simulink model "Linearization2"  (R2022a)
settings: Solver=VariableStepAuto  StartTime=0.0  StopTime=10.0  RelTol=1e-3
undefined symbols (not defined in the file): Aactuator, ac, AeroCoeff, ControlAllocation, DUmax, DUmin, EngineTable, F, fcs, ft, g, hground, IC, kg, LandingGear, Light, LPmethod, m, MIL, Mode_deflection_aileron, Mode_deflection_elevator, Mode_deflection_rudder, Mode_deflection_TVC_y, Mode_deflection_TVC_z, N, Ninv_2nozzle, Ninv_no_nozzle, PIController, s, Sensor, slug, state0, sysID_DAQ, sysID_OBES, Umax_2nozzle, Umax_no_nozzle, Umin_2nozzle, Umin_no_nozzle, WMM2020
libraries: aerolibconvert2 x19, slpidlib x6, simulink x6, sharedutil x4, aerolibatmos2 x3, aerolibwind2 x3, aerolibbdyn x3, aerolibgravity2 x2, sharedtransform x1
(part 8 of 9)

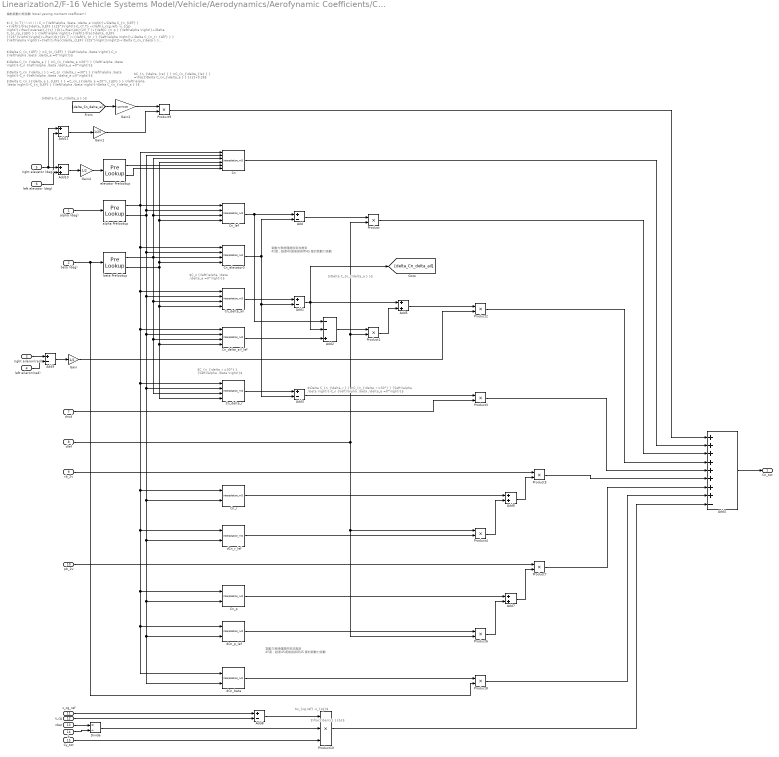
== system Linearization2/F-16 Vehicle Systems Model/Vehicle/Aerodynamics/Aerofynamic Coefficients/CnT ==
  note: $\Delta C_{n_{\delta_a } }$
  note: 氣動力表格僅提供到攻角到
      | 45度，超過45度後皆採用45
      | 度的氣動力係數
  note: 氣動力表格僅提供到攻角到
      | 45度，超過45度後皆採用45
      | 度的氣動力係數
  note: $C_n {\left(\alpha ,\beta ,\delta_e =0°\right)}$
  note: $C_{n_{\delta_r =30°} } {\left(\alpha ,\beta \right)}$
  note: $\Delta C_{n_{\delta_r } } =C_{n_{\delta_r =30°} } {\left(\alpha ,\beta \right)}-C_n {\left(\alpha ,\beta ,\delta_e =0°\right)}$
  note: $x_{cg,ref} -x_{cg}$
  note: $\frac{\bar{c} }{b}$
  note: $\Delta C_{n_{\delta_a } } =C_{n_{\delta_a =20°} } {\left(\alpha ,\beta \right)}-C_n {\left(\alpha ,\beta ,\delta_e =0°\right)}$
  note: $\Delta C_{n_{\delta_r } } =C_{n_{\delta_r =30°} } {\left(\alpha ,\beta \right)}-C_n {\left(\alpha ,\beta ,\delta_e =0°\right)}$
  note: $\ C_{n,T} \ \ =\ \ \ \ C_n {\left(\alpha ,\beta ,\delta_e \right)}+\Delta C_{n_{LEF} } ∙{\left(1-\frac{\delta_{LEF} }{25°}\right)}-C_{Y,T} ∙{\left(x_{cg,ref} -x_{cg} \right)}∙\frac{\overset{-}{c} }{b}+\frac{pb}{2V_T }∙{\left[C_{n_p } {\left(\alpha \right)}+\Delta C_{n_{p_{LEF} } } {\left(\alpha \right)}∙{\left(1-\frac{\delta_{LEF} }{25°}\right)}\right]}+\frac{rb}{2V_T }∙{\left[C_{n_r } {\left(\alpha \right)}+\Delta C_{n_{r_{LEF} } } {\left(\alpha \right)}∙{\left(1-\frac{\delta_{LEF} }{25°}\right)}\right]}+\Delta C_{n_{\beta } } {\left(\alpha \right)}∙\beta +\Delta C_{n_{\delta_r } } ∙{\left(\frac{\delta_r }{30°}\right)}+\frac{{\left[\Delta C_{n_{\delta_a } } +\Delta C_{n_{{\delta_a }_{LEF} } } ∙{\left(1-\frac{\delta_{LEF} }{25°}\right)}\right]}}{2}∙{\left(\frac{\delta_{ra} }{20°}\right)}-\frac{{\left[\Delta C_{n_{\delta_a } } +\Delta C_{n_{{\delta_a }_{LEF} } } ∙{\left(1-\frac{\delta_{LEF} }{25°}\right)}\right]}}{2}∙{\left(\frac{\delta_{la} }{20°}\right)}+C_{n_{\delta_{re} } } ∙{\left(\frac{\delta_{re} }{30°}\right)}-C_{n_{\delta_{le} } } ∙{\left(\frac{\delta_{le} }{30°}\right)}$
  note: $\Delta C_{n_{LEF} } =C_{n_{LEF} } {\left(\alpha ,\beta \right)}-C_n {\left(\alpha ,\beta ,\delta_e =0°\right)}$
  note: 偏航氣動力矩係數 (total yawing moment coefficient)：
  note: $\Delta C_{n_{{\delta_a }_{LEF} } } =C_{n_{{\delta_a =20°}_{LEF} } } {\left(\alpha ,\beta \right)}-C_{n_{LEF} } {\left(\alpha ,\beta \right)}-\Delta C_{n_{\delta_a } }$
  note: $\Delta C_{n_{\delta_a } }$
  note: $C_{n_{\delta_{re} } } =C_{n_{\delta_{le} } } =\frac{\Delta C_{n_{\delta_a } } }{2}∙0.26$
  alpha (deg) : Inport
  beta (deg) : Inport  Port=2
  right aileron(rad) : Inport  Port=3
  left aileron(rad) : Inport  Port=4
  "right elevator (deg) " : Inport  Port=5
  left elevator (deg) : Inport  Port=6
  drud : Inport  Port=7
  dlef : Inport  Port=8
  rb_2v : Inport  Port=9
  pb_2v : Inport  Port=10
  x_cg_ref : Inport  Port=11
  x_cg : Inport  Port=12
  cbar : Inport  Port=13
  b : Inport  Port=14
  Cy_tot : Inport  Port=15
  Add{,1,3,8..9,11} (6 alike) : Sum  Inputs=+-
  Add{5..7,10} (4 alike) : Sum
  Add2 : Sum  Inputs=--+
  Add4 : Sum  Inputs=++++++++-
  Cn : Interpolation_n-D  NumberOfTableDimensions=3  Table=AeroCoeff.Cn
      settings: InputPortMap=u0,u1,u2,u3,u4,u5
  Cn_delta_ail : Interpolation_n-D  Table=AeroCoeff.Cn_delta_ail
  Cn_delta_ail_lef : Interpolation_n-D  Table=AeroCoeff.Cn_delta_ail_lef
  Cn_delta_r : Interpolation_n-D  Table=AeroCoeff.Cn_delta_r
  Cn_elevator0 : Interpolation_n-D  Table=AeroCoeff.Cn_elevator0
  Cn_lef : Interpolation_n-D  Table=AeroCoeff.Cn_lef
  Cn_p : Interpolation_n-D  NumberOfTableDimensions=1  Table=AeroCoeff.Cn_p
      settings: InputPortMap=u0,u1
  Cn_r : Interpolation_n-D  NumberOfTableDimensions=1  Table=AeroCoeff.Cn_r
      settings: InputPortMap=u0,u1
  Divide : Product  Inputs=*/
  Gain : Gain  Gain=1/2
  Gain1 : Gain  Gain=1/25
  Gain2 : Gain  Gain=(1/2)*0.26
  Gain4 : Gain  Gain=1/2
  Product{,1..9} (10 alike) : Product
  Product10 : Product  Inputs=3
  alpha Prelookup : PreLookup  BreakpointsData=AeroCoeff.alpha_prelookup  IndexSearchMethod=Linear search  BeginIndexSearchUsingPreviousIndexResult=on  DiagnosticForOutOfRangeInput=Warning
  beta Prelookup : PreLookup  BreakpointsData=AeroCoeff.beta_prelookup  IndexSearchMethod=Linear search  BeginIndexSearchUsingPreviousIndexResult=on  DiagnosticForOutOfRangeInput=Warning
  dCn_beta : Interpolation_n-D  NumberOfTableDimensions=1  Table=AeroCoeff.dCn_beta
      settings: InputPortMap=u0,u1
  dCn_p_lef : Interpolation_n-D  NumberOfTableDimensions=1  Table=AeroCoeff.dCn_p_lef
      settings: InputPortMap=u0,u1
  dCn_r_lef : Interpolation_n-D  NumberOfTableDimensions=1  Table=AeroCoeff.dCn_r_lef
      settings: InputPortMap=u0,u1
  elevator Prelookup : PreLookup  BreakpointsData=AeroCoeff.elevator_prelookup1  IndexSearchMethod=Linear search  BeginIndexSearchUsingPreviousIndexResult=on  DiagnosticForOutOfRangeInput=Warning
  Cn_tot : Outport  VectorParamsAs1DForOutWhenUnconnected=off
  wires:
  alpha Prelookup/1 -> Cn/1, dCn_p_lef/1, dCn_beta/1, Cn_p/1, dCn_r_lef/1, Cn_r/1, Cn_delta_r/1, Cn_delta_ail_lef/1, Cn_delta_ail/1, Cn_elevator0/1, Cn_lef/1
  Add1/1 -> Add5/1, [delta_Cn_delta_ail], Add2/2
  Cn_elevator0/1 -> Add3/2, Add1/2, Add/2
  alpha Prelookup/2 -> Cn/2, Cn_lef/2, dCn_p_lef/2, dCn_beta/2, Cn_p/2, dCn_r_lef/2, Cn_r/2, Cn_delta_r/2, Cn_delta_ail_lef/2, Cn_delta_ail/2, Cn_elevator0/2
  elevator Prelookup/1 -> Cn/5
  Add6/1 -> Product5/2
  beta Prelookup/2 -> Cn_delta_r/4, Cn_delta_ail_lef/4, Cn_delta_ail/4, Cn/4, Cn_lef/4, Cn_elevator0/4
  Cn_r/1 -> Add6/1
  Cn_delta_ail_lef/1 -> Add2/3
  pb_2v/1 -> Product7/1
  Add5/1 -> Product2/1
  Cn_lef/1 -> Add2/1, Add/1
  Add4/1 -> Cn_tot/1
  Add7/1 -> Product7/2
  beta (deg)/1 -> beta Prelookup/1, Product8/2
  rb_2v/1 -> Product5/1
  Product10/1 -> Add4/9
  Add/1 -> Product/1
  x_cg/1 -> Add8/2
  alpha (deg)/1 -> alpha Prelookup/1
  b/1 -> Divide/2
  dCn_r_lef/1 -> Product4/2
  drud/1 -> Product3/2
  dCn_beta/1 -> Product8/1
  Product4/1 -> Add6/2
  Divide/1 -> Product10/2
  Product3/1 -> Add4/5
  x_cg_ref/1 -> Add8/1
  Cn_p/1 -> Add7/1
  dCn_p_lef/1 -> Product6/1
  Product8/1 -> Add4/8
  elevator Prelookup/2 -> Cn/6
  Cn_delta_r/1 -> Add3/1
  Product6/1 -> Add7/2
  Cy_tot/1 -> Product10/3
  Product7/1 -> Add4/7
  Product5/1 -> Add4/6
  Add2/1 -> Product1/1
  beta Prelookup/1 -> Cn_delta_r/3, Cn_delta_ail_lef/3, Cn_delta_ail/3, Cn/3, Cn_lef/3, Cn_elevator0/3
  Product2/1 -> Add4/4
  Cn/1 -> Add4/2
  Cn_delta_ail/1 -> Add1/1
  Add3/1 -> Product3/1
  dlef/1 -> Product6/2, Product4/1, Product/2, Product1/2
  Product/1 -> Add4/3
  Product1/1 -> Add5/2
  cbar/1 -> Divide/1
  Add8/1 -> Product10/1
  right aileron(rad)/1 -> Add9/1
  left aileron(rad)/1 -> Add9/2
  Add9/1 -> Gain/1
  Gain/1 -> Product2/2
  Add10/1 -> Gain4/1
  [delta_Cn_delta_ail] -> Gain2/1
  Gain1/1 -> Product9/2
  Gain2/1 -> Product9/1
  Product9/1 -> Add4/1
  "right elevator (deg) "/1 -> Add11/1, Add10/1
  left elevator (deg)/1 -> Add11/2, Add10/2
  Add11/1 -> Gain1/1
  Gain4/1 -> elevator Prelookup/1

== system Linearization2/F-16 Vehicle Systems Model/Vehicle/Aerodynamics/Aerofynamic Coefficients/Ground Effects ==
  alpha (deg) : Inport
  beta(deg) : Inport  Port=2
  h_AGL : Inport  Port=3
  Coeff : Outport

== system Linearization2/F-16 Vehicle Systems Model/Vehicle/Aerodynamics/Aerofynamic Coefficients/Landing Gear Effects ==
  alpha (deg) : Inport
  beta(deg) : Inport  Port=2
  Landing Gear Angle : Inport  Port=3
  Coeff : Outport

== system Linearization2/F-16 Vehicle Systems Model/Vehicle/LandingGear GroundReaction/L Main Gear Geometry Forces and Moments/Calc Gear Force and Pos ==
  note: 註:令[ XcB YcB ZcB ] = [ 0 0 0 ]
  note: 詹庭宇:此Block正負號為+---
  note: $∆z_g^B$
  note: $∆z_g^b =z_g^b -z_g^{b^{\prime } } =z_g^b -\frac{z_r^E -z_c^E -C_{31} {\left(x_g^b -x_c^b \right)}-C_{32} {\left(y_g^b -y_c^b \right)}}{C_{33} }$
  note: $z_r^E =z_c^E +C_{31} {\left(x_g^b -x_c^b \right)}+C_{32} {\left(y_g^b -y_c^b \right)}+C_{33} \cdot z_g^{b^{\prime } }$
  note: $z_g^E =z_c^E +C_{31} {\left(x_g^b -x_c^b \right)}+C_{32} {\left(y_g^b -y_c^b \right)}+C_{33} {\left(z_g^b -z_c^b \right)}$
  note: $p^E ={\left[C\right]}{\left(p^b -p_c^b \right)}+p_c^E$
  note: $\left(p^E -p_c^E \right)={\left[C\right]}{\left(p^b -p_c^b \right)}$
  note: 定義：
      | 慣性座標+Z軸朝下
      | 體座標+Z軸朝下
  WOW : Inport
  ZrL : Inport  Port=2
  Xg : Inport  Port=3
  ZcL : Inport  Port=4
  DCM_eb : Inport  Port=5
  Constant : Constant  Value=0
  Demux1 : Demux  Outputs=3
  Demux2 : Demux  Outputs=3
  RangeLimit : Saturate  UpperLimit=LandingGear.LM.CmprsRangeLimitUpper  LowerLimit=LandingGear.LM.CmprsRangeLimitLower
  Subsystem : Subsystem
  Sum1 : Sum  Inputs=+---
  Sum2 : Sum  Inputs=+-
  Switch : Switch  Criteria=u2 ~= 0  Threshold=243  SaturateOnIntegerOverflow=off  InputSameDT=off
  compression : Product  Inputs=*/  RndMeth=Zero
  get_row3 : Selector  NumberOfDimensions=2  InputPortWidth=3  IndexOptions=Index vector (dialog),Select all  Indices=3,-1  OutputSizes=1
  prod1 : Product  RndMeth=Zero
  prod2 : Product  RndMeth=Zero
  dZ_strut : Outport
  Fn_strut : Outport  Port=2
  ZgB_prime : Outport  Port=3
  wires:
  ZrL/1 -> Sum1/1
  DCM_eb/1 -> get_row3/1
  get_row3/1 -> Demux1/1  "C3"
  Demux1/1 -> prod1/2  "C31"
  Demux1/2 -> prod2/2  "C32"
  Demux2/1 -> prod1/1  "XgB-XcB"
  Demux2/2 -> prod2/1  "YgB-YcB"
  prod1/1 -> Sum1/3
  prod2/1 -> Sum1/4
  Demux1/3 -> compression/2, Subsystem/2(C33)  "C33"
  Subsystem/2(Fn_strut) -> Fn_strut/1
  compression/1 -> Sum2/2, ZgB_prime/1
  ZcL/1 -> Sum1/2
  Xg/1 -> Demux2/1
  Sum1/1 -> compression/1  "Strut_dZnum"
  Demux2/3 -> Sum2/1  "ZgB-ZcB"
  Subsystem/1(dZ_strut) -> dZ_strut/1
  RangeLimit/1 -> Subsystem/1(deltaZgB)
  Switch/1 -> RangeLimit/1
  Sum2/1 -> Switch/1  "T command"
  WOW/1 -> Switch/2
  Constant/1 -> Switch/3  "T command"

== system Linearization2/F-16 Vehicle Systems Model/Vehicle/LandingGear GroundReaction/L Main Gear Geometry Forces and Moments/GenerateGroundFM ==
  note: 正負號可能相反
  note: 慣性座標轉至體座標的旋轉矩陣
  note: 詹庭宇:拿掉/忽略輪胎側向力模型，Fy=0
  note: 詹庭宇:拿掉/忽略輪胎側向力模型，Fy=0
  GearLoc : Inport
  Fn_strut : Inport  Port=2
  ZgB_prime : Inport  Port=3
  DCM_be : Inport  Port=4
  plant : Inport  Port=5
  Enable : EnablePort
  Constant : Constant  Value=0
  Constant1 : Constant  Value=[0 0 0]
  Demux : Demux  Outputs=3
  Forces and distances to LMN : Subsystem
  Gear Local Force vector : Concatenate  NumInputs=3  Mode=Multidimensional array
  LocMatrix1 : Subsystem
  Local Forces to Body Axes : Product  Multiplication=Matrix(*)  InputSameDT=on  SaturateOnIntegerOverflow=on  OutDataTypeStr=Inherit: Same as first input
  Manual Switch : ManualSwitch  CurrentSetting=0
  Moments about CG due to Forces : aerolibbdyn/Moments about CG  due to Forces
      settings: SourceProductBaseCode=AE
  Mux1 : Mux  Inputs=2
  Mux2 : Mux  Inputs=3
  Rotation Speed(TVC ON) : Subsystem
  Terminator : Terminator
  FM : Outport
  wires:
  DCM_be/1 -> Local Forces to Body Axes/1
  Mux1/1 -> FM/1
  Local Forces to Body Axes/1 -> Moments about CG due to Forces/1, Forces and distances to LMN/1(Fb)
  Gear Local Force vector/1 -> Local Forces to Body Axes/2, Mux1/1
  Constant/1 -> Gear Local Force vector/2
  ZgB_prime/1 -> Mux2/3, LocMatrix1/2(ZgB_prime)
  Forces and distances to LMN/1(LMNe) -> Manual Switch/1
  Manual Switch/1 -> Mux1/2
  Moments about CG due to Forces/1 -> Manual Switch/2
  Constant1/1 -> Moments about CG due to Forces/2
  LocMatrix1/1(A) -> Forces and distances to LMN/2(Xg_gnd)
  Demux/1 -> Mux2/1
  Demux/3 -> Terminator/1
  GearLoc/1 -> Demux/1, LocMatrix1/1(XgB)
  Mux2/1 -> Moments about CG due to Forces/3
  Demux/2 -> Mux2/2
  plant/1 -> Rotation Speed(TVC ON)/2(PlantData)
  Fn_strut/1 -> Gear Local Force vector/3, Rotation Speed(TVC ON)/1(friction)
  Rotation Speed(TVC ON)/1(output) -> Gear Local Force vector/1

== system Linearization2/F-16 Vehicle Systems Model/Vehicle/LandingGear GroundReaction/Nose Gear Geometry Forces and Moments/Calc Gear Force and Pos ==
  note: 註:令[ XcB YcB ZcB ] = [ 0 0 0 ]
  note: 詹庭宇:此Block正負號為+---
  note: $∆z_g^B$
  note: $∆z_g^b =z_g^b -z_g^{b^{\prime } } =z_g^b -\frac{z_r^E -z_c^E -C_{31} {\left(x_g^b -x_c^b \right)}-C_{32} {\left(y_g^b -y_c^b \right)}}{C_{33} }$
  note: $z_r^E =z_c^E +C_{31} {\left(x_g^b -x_c^b \right)}+C_{32} {\left(y_g^b -y_c^b \right)}+C_{33} \cdot z_g^{b^{\prime } }$
  note: $z_g^E =z_c^E +C_{31} {\left(x_g^b -x_c^b \right)}+C_{32} {\left(y_g^b -y_c^b \right)}+C_{33} {\left(z_g^b -z_c^b \right)}$
  note: $p^E ={\left[C\right]}{\left(p^b -p_c^b \right)}+p_c^E$
  note: $\left(p^E -p_c^E \right)={\left[C\right]}{\left(p^b -p_c^b \right)}$
  note: 定義：
      | 慣性座標+Z軸朝下
      | 體座標+Z軸朝下
  WOW : Inport
  ZrL : Inport  Port=2
  Xg : Inport  Port=3
  ZcL : Inport  Port=4
  DCM_eb : Inport  Port=5
  Constant : Constant  Value=0
  Demux1 : Demux  Outputs=3
  Demux2 : Demux  Outputs=3
  RangeLimit : Saturate  UpperLimit=LandingGear.Nose.CmprsRangeLimitUpper  LowerLimit=LandingGear.Nose.CmprsRangeLimitLower
  Subsystem : Subsystem
  Sum1 : Sum  Inputs=+---
  Sum2 : Sum  Inputs=+-
  Switch : Switch  Criteria=u2 ~= 0  Threshold=243  SaturateOnIntegerOverflow=off  InputSameDT=off
  compression : Product  Inputs=*/  RndMeth=Zero
  get_row3 : Selector  NumberOfDimensions=2  InputPortWidth=3  IndexOptions=Index vector (dialog),Select all  Indices=3,-1  OutputSizes=1
  prod1 : Product  RndMeth=Zero
  prod2 : Product  RndMeth=Zero
  dZ_strut : Outport
  Fn_strut : Outport  Port=2
  ZgB_prime : Outport  Port=3
  wires:
  ZrL/1 -> Sum1/1
  DCM_eb/1 -> get_row3/1
  get_row3/1 -> Demux1/1  "C3"
  Demux1/1 -> prod1/2  "C31"
  Demux1/2 -> prod2/2  "C32"
  Demux2/1 -> prod1/1  "XgB-XcB"
  Demux2/2 -> prod2/1  "YgB-YcB"
  prod1/1 -> Sum1/3
  prod2/1 -> Sum1/4
  Demux1/3 -> compression/2, Subsystem/2(C33)  "C33"
  Subsystem/2(Fn_strut) -> Fn_strut/1
  compression/1 -> Sum2/2, ZgB_prime/1
  ZcL/1 -> Sum1/2
  Xg/1 -> Demux2/1
  Sum1/1 -> compression/1  "Strut_dZnum"
  Demux2/3 -> Sum2/1  "ZgB-ZcB"
  Subsystem/1(dZ_strut) -> dZ_strut/1
  RangeLimit/1 -> Subsystem/1(deltaZgB)
  Switch/1 -> RangeLimit/1
  Sum2/1 -> Switch/1  "T command"
  WOW/1 -> Switch/2
  Constant/1 -> Switch/3  "T command"

== system Linearization2/F-16 Vehicle Systems Model/Vehicle/LandingGear GroundReaction/Nose Gear Geometry Forces and Moments/GenerateGroundFM ==
  note: 正負號可能相反
  note: 慣性座標轉至體座標的旋轉矩陣
  note: 詹庭宇:拿掉/忽略輪胎側向力模型，Fy=0
  note: 詹庭宇:拿掉/忽略輪胎側向力模型，Fy=0
  GearLoc : Inport
  Fn_strut : Inport  Port=2
  ZgB_prime : Inport  Port=3
  DCM_be : Inport  Port=4
  plant : Inport  Port=5
  Enable : EnablePort
  Constant : Constant  Value=0
  Constant1 : Constant  Value=[0 0 0]
  Demux : Demux  Outputs=3
  Forces and distances to LMN : Subsystem
  Gear Local Force vector : Concatenate  NumInputs=3  Mode=Multidimensional array
  LocMatrix1 : Subsystem
  Local Forces to Body Axes : Product  Multiplication=Matrix(*)  InputSameDT=on  SaturateOnIntegerOverflow=on  OutDataTypeStr=Inherit: Same as first input
  Manual Switch : ManualSwitch  CurrentSetting=0
  Moments about CG due to Forces : aerolibbdyn/Moments about CG  due to Forces
      settings: SourceProductBaseCode=AE
  Mux1 : Mux  Inputs=2
  Mux2 : Mux  Inputs=3
  Rotation Speed(TVC ON) : Subsystem
  Terminator : Terminator
  FM : Outport
  wires:
  DCM_be/1 -> Local Forces to Body Axes/1
  Mux1/1 -> FM/1
  Local Forces to Body Axes/1 -> Moments about CG due to Forces/1, Forces and distances to LMN/1(Fb)
  Gear Local Force vector/1 -> Local Forces to Body Axes/2, Mux1/1
  Constant/1 -> Gear Local Force vector/2
  ZgB_prime/1 -> Mux2/3, LocMatrix1/2(ZgB_prime)
  Forces and distances to LMN/1(LMNe) -> Manual Switch/1
  Manual Switch/1 -> Mux1/2
  Moments about CG due to Forces/1 -> Manual Switch/2
  Constant1/1 -> Moments about CG due to Forces/2
  LocMatrix1/1(A) -> Forces and distances to LMN/2(Xg_gnd)
  Demux/1 -> Mux2/1
  Demux/3 -> Terminator/1
  GearLoc/1 -> Demux/1, LocMatrix1/1(XgB)
  Mux2/1 -> Moments about CG due to Forces/3
  Demux/2 -> Mux2/2
  plant/1 -> Rotation Speed(TVC ON)/2(PlantData)
  Fn_strut/1 -> Gear Local Force vector/3, Rotation Speed(TVC ON)/1(friction)
  Rotation Speed(TVC ON)/1(output) -> Gear Local Force vector/1

== system Linearization2/F-16 Vehicle Systems Model/Vehicle/LandingGear GroundReaction/R Main Gear Geometry Forces and Moments/Calc Gear Force and Pos ==
  note: 註:令[ XcB YcB ZcB ] = [ 0 0 0 ]
  note: 詹庭宇:此Block正負號為+---
  note: $∆z_g^B$
  note: $∆z_g^b =z_g^b -z_g^{b^{\prime } } =z_g^b -\frac{z_r^E -z_c^E -C_{31} {\left(x_g^b -x_c^b \right)}-C_{32} {\left(y_g^b -y_c^b \right)}}{C_{33} }$
  note: $z_r^E =z_c^E +C_{31} {\left(x_g^b -x_c^b \right)}+C_{32} {\left(y_g^b -y_c^b \right)}+C_{33} \cdot z_g^{b^{\prime } }$
  note: $z_g^E =z_c^E +C_{31} {\left(x_g^b -x_c^b \right)}+C_{32} {\left(y_g^b -y_c^b \right)}+C_{33} {\left(z_g^b -z_c^b \right)}$
  note: $p^E ={\left[C\right]}{\left(p^b -p_c^b \right)}+p_c^E$
  note: $\left(p^E -p_c^E \right)={\left[C\right]}{\left(p^b -p_c^b \right)}$
  note: 定義：
      | 慣性座標+Z軸朝下
      | 體座標+Z軸朝下
  WOW : Inport
  ZrL : Inport  Port=2
  Xg : Inport  Port=3
  ZcL : Inport  Port=4
  DCM_eb : Inport  Port=5
  Constant : Constant  Value=0
  Demux1 : Demux  Outputs=3
  Demux2 : Demux  Outputs=3
  RangeLimit : Saturate  UpperLimit=LandingGear.RM.CmprsRangeLimitUpper  LowerLimit=LandingGear.RM.CmprsRangeLimitLower
  Subsystem : Subsystem
  Sum1 : Sum  Inputs=+---
  Sum2 : Sum  Inputs=+-
  Switch : Switch  Criteria=u2 ~= 0  Threshold=243  SaturateOnIntegerOverflow=off  InputSameDT=off
  compression : Product  Inputs=*/  RndMeth=Zero
  get_row3 : Selector  NumberOfDimensions=2  InputPortWidth=3  IndexOptions=Index vector (dialog),Select all  Indices=3,-1  OutputSizes=1
  prod1 : Product  RndMeth=Zero
  prod2 : Product  RndMeth=Zero
  dZ_strut : Outport
  Fn_strut : Outport  Port=2
  ZgB_prime : Outport  Port=3
  wires:
  ZrL/1 -> Sum1/1
  DCM_eb/1 -> get_row3/1
  get_row3/1 -> Demux1/1  "C3"
  Demux1/1 -> prod1/2  "C31"
  Demux1/2 -> prod2/2  "C32"
  Demux2/1 -> prod1/1  "XgB-XcB"
  Demux2/2 -> prod2/1  "YgB-YcB"
  prod1/1 -> Sum1/3
  prod2/1 -> Sum1/4
  Demux1/3 -> compression/2, Subsystem/2(C33)  "C33"
  Subsystem/2(Fn_strut) -> Fn_strut/1
  compression/1 -> Sum2/2, ZgB_prime/1
  ZcL/1 -> Sum1/2
  Xg/1 -> Demux2/1
  Sum1/1 -> compression/1  "Strut_dZnum"
  Demux2/3 -> Sum2/1  "ZgB-ZcB"
  Subsystem/1(dZ_strut) -> dZ_strut/1
  RangeLimit/1 -> Subsystem/1(deltaZgB)
  Switch/1 -> RangeLimit/1
  Sum2/1 -> Switch/1  "T command"
  WOW/1 -> Switch/2
  Constant/1 -> Switch/3  "T command"

== system Linearization2/F-16 Vehicle Systems Model/Vehicle/LandingGear GroundReaction/R Main Gear Geometry Forces and Moments/GenerateGroundFM ==
  note: 正負號可能相反
  note: 慣性座標轉至體座標的旋轉矩陣
  note: 詹庭宇:拿掉/忽略輪胎側向力模型，Fy=0
  note: 詹庭宇:拿掉/忽略輪胎側向力模型，Fy=0
  GearLoc : Inport
  Fn_strut : Inport  Port=2
  ZgB_prime : Inport  Port=3
  DCM_be : Inport  Port=4
  plant : Inport  Port=5
  Enable : EnablePort
  Constant : Constant  Value=0
  Constant1 : Constant  Value=[0 0 0]
  Demux : Demux  Outputs=3
  Forces and distances to LMN : Subsystem
  Gear Local Force vector : Concatenate  NumInputs=3  Mode=Multidimensional array
  LocMatrix1 : Subsystem
  Local Forces to Body Axes : Product  Multiplication=Matrix(*)  InputSameDT=on  SaturateOnIntegerOverflow=on  OutDataTypeStr=Inherit: Same as first input
  Manual Switch : ManualSwitch  CurrentSetting=0
  Moments about CG due to Forces : aerolibbdyn/Moments about CG  due to Forces
      settings: SourceProductBaseCode=AE
  Mux1 : Mux  Inputs=2
  Mux2 : Mux  Inputs=3
  Rotation Speed(TVC ON) : Subsystem
  Terminator : Terminator
  FM : Outport
  wires:
  DCM_be/1 -> Local Forces to Body Axes/1
  Mux1/1 -> FM/1
  Local Forces to Body Axes/1 -> Moments about CG due to Forces/1, Forces and distances to LMN/1(Fb)
  Gear Local Force vector/1 -> Local Forces to Body Axes/2, Mux1/1
  Constant/1 -> Gear Local Force vector/2
  ZgB_prime/1 -> Mux2/3, LocMatrix1/2(ZgB_prime)
  Forces and distances to LMN/1(LMNe) -> Manual Switch/1
  Manual Switch/1 -> Mux1/2
  Moments about CG due to Forces/1 -> Manual Switch/2
  Constant1/1 -> Moments about CG due to Forces/2
  LocMatrix1/1(A) -> Forces and distances to LMN/2(Xg_gnd)
  Demux/1 -> Mux2/1
  Demux/3 -> Terminator/1
  GearLoc/1 -> Demux/1, LocMatrix1/1(XgB)
  Mux2/1 -> Moments about CG due to Forces/3
  Demux/2 -> Mux2/2
  plant/1 -> Rotation Speed(TVC ON)/2(PlantData)
  Fn_strut/1 -> Gear Local Force vector/3, Rotation Speed(TVC ON)/1(friction)
  Rotation Speed(TVC ON)/1(output) -> Gear Local Force vector/1

== system Linearization2/F-16 Vehicle Systems Model/Vehicle/Propulsion/Afterburning Turbofan Jet Engine/If Action Subsystem ==
  note: Pow_max
      |
      | Pow_min
      |
      | T_idle
      |
      | T_mil
      |
      | T_max
  "input " : Inport
  Action Port : ActionPort
  Add : Sum
  Add1 : Sum  Inputs=-+
  Demux : Demux  Outputs=5
  Divide : Product  Inputs=**
  Gain : Gain  Gain=1/50
  Terminator : Terminator
  Terminator1 : Terminator
  T_max1 : Outport  VectorParamsAs1DForOutWhenUnconnected=off
  wires:
  Demux/3 -> Add1/1, Add/1
  Demux/4 -> Add1/2
  Add1/1 -> Divide/2
  Gain/1 -> Divide/1
  Divide/1 -> Add/2
  Add/1 -> T_max1/1
  "input "/1 -> Demux/1
  Demux/1 -> Gain/1
  Demux/2 -> Terminator/1
  Demux/5 -> Terminator1/1

== system Linearization2/F-16 Vehicle Systems Model/Vehicle/Propulsion/Afterburning Turbofan Jet Engine/If Action Subsystem1 ==
  note: Pow_max
      |
      | Pow_min
      |
      | T_idle
      |
      | T_mil
      |
      | T_max
  "input " : Inport
  Action Port : ActionPort
  Add : Sum
  Add1 : Sum  Inputs=-+
  Add2 : Sum  Inputs=-+
  Constant : Constant  Value=50
  Demux : Demux  Outputs=5
  Gain : Gain  Gain=1/50
  Product : Product
  Terminator : Terminator
  Terminator1 : Terminator
  T_max1 : Outport  VectorParamsAs1DForOutWhenUnconnected=off
  wires:
  "input "/1 -> Demux/1
  Demux/4 -> Add/2, Add1/1
  Demux/5 -> Add1/2
  Demux/1 -> Add2/2
  Constant/1 -> Add2/1
  Add2/1 -> Gain/1
  Add1/1 -> Product/2
  Gain/1 -> Product/1
  Product/1 -> Add/1
  Add/1 -> T_max1/1
  Demux/3 -> Terminator1/1
  Demux/2 -> Terminator/1

== system Linearization2/F-16 Vehicle Systems Model/Vehicle/Propulsion/Afterburning Turbofan Jet Engine/If Action Subsystem2 ==
  note: Pow_max
      |
      | Pow_min
      |
      | T_idle
      |
      | T_mil
      |
      | T_max
  "input " : Inport
  Action Port : ActionPort
  Add : Sum
  Add1 : Sum  Inputs=-+
  Demux : Demux  Outputs=5
  Divide : Product  Inputs=**
  Gain : Gain  Gain=1/50
  Terminator : Terminator
  Terminator1 : Terminator
  T_min : Outport  VectorParamsAs1DForOutWhenUnconnected=off
  wires:
  Demux/3 -> Add1/1, Add/1
  Demux/4 -> Add1/2
  Add1/1 -> Divide/2
  Gain/1 -> Divide/1
  Divide/1 -> Add/2
  Add/1 -> T_min/1
  "input "/1 -> Demux/1
  Demux/2 -> Gain/1
  Demux/5 -> Terminator1/1
  Demux/1 -> Terminator/1

== system Linearization2/F-16 Vehicle Systems Model/Vehicle/Propulsion/Afterburning Turbofan Jet Engine/If Action Subsystem3 ==
  note: Pow_max
      |
      | Pow_min
      |
      | T_idle
      |
      | T_mil
      |
      | T_max
  "input " : Inport
  Action Port : ActionPort
  Add : Sum
  Add1 : Sum  Inputs=-+
  Add2 : Sum  Inputs=-+
  Constant : Constant  Value=50
  Demux : Demux  Outputs=5
  Gain : Gain  Gain=1/50
  Product : Product
  Terminator : Terminator
  Terminator1 : Terminator
  T_min : Outport  VectorParamsAs1DForOutWhenUnconnected=off
  wires:
  "input "/1 -> Demux/1
  Demux/4 -> Add/2, Add1/1
  Demux/5 -> Add1/2
  Constant/1 -> Add2/1
  Add2/1 -> Gain/1
  Add1/1 -> Product/2
  Gain/1 -> Product/1
  Product/1 -> Add/1
  Add/1 -> T_min/1
  Demux/3 -> Terminator1/1
  Demux/2 -> Add2/2
  Demux/1 -> Terminator/1

== system Linearization2/F-16 Vehicle Systems Model/Vehicle/Propulsion/Afterburning Turbofan Jet Engine/If Action Subsystem4 ==
  In1 : Inport
  Action Port : ActionPort
  Out1 : Outport
  wires:
  In1/1 -> Out1/1

== system Linearization2/F-16 Vehicle Systems Model/Vehicle/Propulsion/Afterburning Turbofan Jet Engine/If Action Subsystem5 ==
  In1 : Inport
  Action Port : ActionPort
  Out1 : Outport
  wires:
  In1/1 -> Out1/1

== system Linearization2/F-16 Vehicle Systems Model/Vehicle/Propulsion/Afterburning Turbofan Jet Engine/If Action Subsystem6 ==
  In1 : Inport
  Action Port : ActionPort
  Out1 : Outport
  wires:
  In1/1 -> Out1/1

== system Linearization2/F-16 Vehicle Systems Model/Vehicle/Propulsion(two_nozzles)/Afterburning Turbofan Jet Engine/If Action Subsystem ==
  note: Pow_max
      |
      | Pow_min
      |
      | T_idle
      |
      | T_mil
      |
      | T_max
  "input " : Inport
  Action Port : ActionPort  ActionPortLabel=if(u1<50)
  Add : Sum
  Add1 : Sum  Inputs=-+
  Demux : Demux  Outputs=5
  Divide : Product  Inputs=**
  Gain : Gain  Gain=1/50
  Terminator : Terminator
  Terminator1 : Terminator
  T_max1 : Outport  VectorParamsAs1DForOutWhenUnconnected=off
  wires:
  Demux/3 -> Add1/1, Add/1
  Demux/4 -> Add1/2
  Add1/1 -> Divide/2
  Gain/1 -> Divide/1
  Divide/1 -> Add/2
  Add/1 -> T_max1/1
  "input "/1 -> Demux/1
  Demux/1 -> Gain/1
  Demux/2 -> Terminator/1
  Demux/5 -> Terminator1/1

== system Linearization2/F-16 Vehicle Systems Model/Vehicle/Propulsion(two_nozzles)/Afterburning Turbofan Jet Engine/If Action Subsystem1 ==
  note: Pow_max
      |
      | Pow_min
      |
      | T_idle
      |
      | T_mil
      |
      | T_max
  "input " : Inport
  Action Port : ActionPort  ActionPortLabel=elseif(u1>=50)
  Add : Sum
  Add1 : Sum  Inputs=-+
  Add2 : Sum  Inputs=-+
  Constant : Constant  Value=50
  Demux : Demux  Outputs=5
  Gain : Gain  Gain=1/50
  Product : Product
  Terminator : Terminator
  Terminator1 : Terminator
  T_max1 : Outport  VectorParamsAs1DForOutWhenUnconnected=off
  wires:
  "input "/1 -> Demux/1
  Demux/4 -> Add/2, Add1/1
  Demux/5 -> Add1/2
  Demux/1 -> Add2/2
  Constant/1 -> Add2/1
  Add2/1 -> Gain/1
  Add1/1 -> Product/2
  Gain/1 -> Product/1
  Product/1 -> Add/1
  Add/1 -> T_max1/1
  Demux/3 -> Terminator1/1
  Demux/2 -> Terminator/1

== system Linearization2/F-16 Vehicle Systems Model/Vehicle/Propulsion(two_nozzles)/Afterburning Turbofan Jet Engine/If Action Subsystem2 ==
  note: Pow_max
      |
      | Pow_min
      |
      | T_idle
      |
      | T_mil
      |
      | T_max
  "input " : Inport
  Action Port : ActionPort  ActionPortLabel=if(u1<50)
  Add : Sum
  Add1 : Sum  Inputs=-+
  Demux : Demux  Outputs=5
  Divide : Product  Inputs=**
  Gain : Gain  Gain=1/50
  Terminator : Terminator
  Terminator1 : Terminator
  T_min : Outport  VectorParamsAs1DForOutWhenUnconnected=off
  wires:
  Demux/3 -> Add1/1, Add/1
  Demux/4 -> Add1/2
  Add1/1 -> Divide/2
  Gain/1 -> Divide/1
  Divide/1 -> Add/2
  Add/1 -> T_min/1
  "input "/1 -> Demux/1
  Demux/2 -> Gain/1
  Demux/5 -> Terminator1/1
  Demux/1 -> Terminator/1

== system Linearization2/F-16 Vehicle Systems Model/Vehicle/Propulsion(two_nozzles)/Afterburning Turbofan Jet Engine/If Action Subsystem3 ==
  note: Pow_max
      |
      | Pow_min
      |
      | T_idle
      |
      | T_mil
      |
      | T_max
  "input " : Inport
  Action Port : ActionPort  ActionPortLabel=elseif(u1>=50)
  Add : Sum
  Add1 : Sum  Inputs=-+
  Add2 : Sum  Inputs=-+
  Constant : Constant  Value=50
  Demux : Demux  Outputs=5
  Gain : Gain  Gain=1/50
  Product : Product
  Terminator : Terminator
  Terminator1 : Terminator
  T_min : Outport  VectorParamsAs1DForOutWhenUnconnected=off
  wires:
  "input "/1 -> Demux/1
  Demux/4 -> Add/2, Add1/1
  Demux/5 -> Add1/2
  Constant/1 -> Add2/1
  Add2/1 -> Gain/1
  Add1/1 -> Product/2
  Gain/1 -> Product/1
  Product/1 -> Add/1
  Add/1 -> T_min/1
  Demux/3 -> Terminator1/1
  Demux/2 -> Add2/2
  Demux/1 -> Terminator/1

== system Linearization2/F-16 Vehicle Systems Model/Vehicle/Propulsion(two_nozzles)/Afterburning Turbofan Jet Engine/If Action Subsystem4 ==
  In1 : Inport
  Action Port : ActionPort  ActionPortLabel=if(u3 == u1)
  Out1 : Outport
  wires:
  In1/1 -> Out1/1

== system Linearization2/F-16 Vehicle Systems Model/Vehicle/Propulsion(two_nozzles)/Afterburning Turbofan Jet Engine/If Action Subsystem5 ==
  In1 : Inport
  Action Port : ActionPort  ActionPortLabel=elseif(u3>u1 & u3<=u2)
  Out1 : Outport
  wires:
  In1/1 -> Out1/1

== system Linearization2/F-16 Vehicle Systems Model/Vehicle/Propulsion(two_nozzles)/Afterburning Turbofan Jet Engine/If Action Subsystem6 ==
  In1 : Inport
  Action Port : ActionPort  ActionPortLabel=else
  Out1 : Outport
  wires:
  In1/1 -> Out1/1

== system Linearization2/F-16 Vehicle Systems Model/Vehicle/LandingGear GroundReaction/L Main Gear Geometry Forces and Moments/Calc Gear Force and Pos/Subsystem ==
  note: 地面正向力(慣性座標)
  note: $N=F_{strut} /C_{33}$
  note: $F_{strut} =K{\left(∆z_g^B \right)}+C{\left(∆{\dot{z} }_g^B \right)}$
      | 支柱上的作用力(體座標)
  note: $∆{\dot{z} }_g^B$
  note: 定義：
      | 慣性座標+Z軸朝下
      | 體座標+Z軸朝下
  deltaZgB : Inport
  C33 : Inport  Port=2
  DampingConstant_N/m/sec1 : Gain  Gain=LandingGear.LM.DampingConstant
  NormalForce : Product  Inputs=*/  RndMeth=Zero
  SpringConstant_N/m1 : Gain  Gain=LandingGear.LM.SpringConstant
  Sum2 : Sum
  Xcmpr_prev : Memory  InheritSampleTime=on
  dCompression : Sum  Inputs=+-
  ground only pushes : Saturate  UpperLimit=inf  LowerLimit=0
  reaction : Gain  Gain=-1
  dZ_strut : Outport
  Fn_strut : Outport  Port=2
  wires:
  deltaZgB/1 -> Xcmpr_prev/1, dCompression/1, SpringConstant_N/m1/1, dZ_strut/1
  dCompression/1 -> DampingConstant_N/m/sec1/1
  DampingConstant_N/m/sec1/1 -> Sum2/2
  SpringConstant_N/m1/1 -> Sum2/1
  Sum2/1 -> NormalForce/1  "Fstrut"
  NormalForce/1 -> ground only pushes/1
  ground only pushes/1 -> reaction/1
  reaction/1 -> Fn_strut/1
  Xcmpr_prev/1 -> dCompression/2
  C33/1 -> NormalForce/2

== system Linearization2/F-16 Vehicle Systems Model/Vehicle/LandingGear GroundReaction/L Main Gear Geometry Forces and Moments/GenerateGroundFM/Forces and distances to LMN ==
  Fb : Inport
  Xg_gnd : Inport  Port=2
  force to moment : Product  Multiplication=Matrix(*)  InputSameDT=on  SaturateOnIntegerOverflow=on  OutDataTypeStr=Inherit: Same as first input
  transpose : Reshape  OutputDimensionality=Row vector (2-D)  OutputDimensions=[1,3]
  transpose1 : Reshape  OutputDimensionality=Column vector (2-D)  OutputDimensions=[1,3]
  LMNe : Outport
  wires:
  Fb/1 -> transpose/1
  transpose/1 -> force to moment/1
  Xg_gnd/1 -> force to moment/2
  force to moment/1 -> transpose1/1
  transpose1/1 -> LMNe/1

== system Linearization2/F-16 Vehicle Systems Model/Vehicle/LandingGear GroundReaction/L Main Gear Geometry Forces and Moments/GenerateGroundFM/LocMatrix1 ==
  note: 正負號可能相反
  note: $z_g^{B^{\prime } }$
  note: $x_g^B$
  note: ${\left\{\begin{array}{c} L_G =Y_G \cdot z_g^{B^{\prime } } -Z_G \cdot y_g^B \\ M_G =Z_G \cdot x_g^B -X_G \cdot z_g^{B^{\prime } } \\ N_G =X_G \cdot y_g^B -Y_G \cdot x_g^B \end{array}\right)}={\left[\begin{array}{ccc} 0 & z_g^{B^{\prime } } & -y_g^B \\ -z_g^{B^{\prime } } & 0 & x_g^B \\ y_g^B & -x_g^B & 0 \end{array}\right]}{\left[\begin{array}{c} X_G \\ Y_G \\ Z_G \end{array}\right]}={\left[\begin{array}{ccc} A_{11} & A_{12} & A_{13} \\ A_{21} & A_{22} & A_{23} \\ A_{31} & A_{32} & A_{33} \end{array}\right]}{\left[\begin{array}{c} X_G \\ Y_G \\ Z_G \end{array}\right]}$
  note: 詹庭宇:HL-20 example建模正負號有誤
  note: $y_g^B$
  note: $z_g^B$
  XgB : Inport
  ZgB_prime : Inport  Port=2
  Create 3x3 Matrix : sharedutil/Create 3x3 Matrix  aMode=aMode
      settings: SourceProductBaseCode=AE,PW,DR,MT,VE
  Demux2 : Demux  Outputs=3
  Terminator1 : Terminator
  inv1 : Gain  Gain=-1
  inv3 : Gain  Gain=-1
  inv4 : Gain  Gain=-1
  zero1 : Constant  Value=0  SampleTime=0
  zero2 : Constant  Value=0  SampleTime=0
  zero3 : Constant  Value=0  SampleTime=0
  A : Outport
  wires:
  XgB/1 -> Demux2/1
  Create 3x3 Matrix/1 -> A/1
  zero1/1 -> Create 3x3 Matrix/1
  Demux2/3 -> Terminator1/1
  ZgB_prime/1 -> Create 3x3 Matrix/2, inv4/1
  zero2/1 -> Create 3x3 Matrix/5
  zero3/1 -> Create 3x3 Matrix/9
  Demux2/2 -> Create 3x3 Matrix/7, inv1/1
  Demux2/1 -> Create 3x3 Matrix/6, inv3/1
  inv1/1 -> Create 3x3 Matrix/3
  inv4/1 -> Create 3x3 Matrix/4
  inv3/1 -> Create 3x3 Matrix/8

== system Linearization2/F-16 Vehicle Systems Model/Vehicle/LandingGear GroundReaction/L Main Gear Geometry Forces and Moments/GenerateGroundFM/Rotation Speed(TVC ON) ==
  friction : Inport
  In Bus Element38 : Inport  Port=2  PortName=PlantData  Element=Vt
  Gain1 : Gain  Gain=0.1
  Gain2 : Gain  Gain=0.5
  Switch : Switch  Threshold=180  SaturateOnIntegerOverflow=off  InputSameDT=off
  output : Outport
  wires:
  In Bus Element38/1 -> Switch/2
  friction/1 -> Gain1/1, Gain2/1
  Switch/1 -> output/1
  Gain2/1 -> Switch/3
  Gain1/1 -> Switch/1

== system Linearization2/F-16 Vehicle Systems Model/Vehicle/LandingGear GroundReaction/Nose Gear Geometry Forces and Moments/Calc Gear Force and Pos/Subsystem ==
  note: 地面正向力(慣性座標)
  note: $N=F_{strut} /C_{33}$
  note: $F_{strut} =K{\left(∆z_g^B \right)}+C{\left(∆{\dot{z} }_g^B \right)}$
      | 支柱上的作用力(體座標)
  note: $∆{\dot{z} }_g^B$
  note: 定義：
      | 慣性座標+Z軸朝下
      | 體座標+Z軸朝下
  deltaZgB : Inport
  C33 : Inport  Port=2
  DampingConstant_N/m/sec1 : Gain  Gain=LandingGear.Nose.DampingConstant
  NormalForce : Product  Inputs=*/  RndMeth=Zero
  SpringConstant_N/m1 : Gain  Gain=LandingGear.Nose.SpringConstant
  Sum2 : Sum
  Xcmpr_prev : Memory  InheritSampleTime=on
  dCompression : Sum  Inputs=+-
  ground only pushes : Saturate  UpperLimit=inf  LowerLimit=0
  reaction : Gain  Gain=-1
  dZ_strut : Outport
  Fn_strut : Outport  Port=2
  wires:
  deltaZgB/1 -> Xcmpr_prev/1, dCompression/1, SpringConstant_N/m1/1, dZ_strut/1
  dCompression/1 -> DampingConstant_N/m/sec1/1
  DampingConstant_N/m/sec1/1 -> Sum2/2
  SpringConstant_N/m1/1 -> Sum2/1
  Sum2/1 -> NormalForce/1  "Fstrut"
  NormalForce/1 -> ground only pushes/1
  ground only pushes/1 -> reaction/1
  reaction/1 -> Fn_strut/1
  Xcmpr_prev/1 -> dCompression/2
  C33/1 -> NormalForce/2

== system Linearization2/F-16 Vehicle Systems Model/Vehicle/LandingGear GroundReaction/Nose Gear Geometry Forces and Moments/GenerateGroundFM/Forces and distances to LMN ==
  Fb : Inport
  Xg_gnd : Inport  Port=2
  force to moment : Product  Multiplication=Matrix(*)  InputSameDT=on  SaturateOnIntegerOverflow=on  OutDataTypeStr=Inherit: Same as first input
  transpose : Reshape  OutputDimensionality=Row vector (2-D)  OutputDimensions=[1,3]
  transpose1 : Reshape  OutputDimensionality=Column vector (2-D)  OutputDimensions=[1,3]
  LMNe : Outport
  wires:
  Fb/1 -> transpose/1
  transpose/1 -> force to moment/1
  Xg_gnd/1 -> force to moment/2
  force to moment/1 -> transpose1/1
  transpose1/1 -> LMNe/1

== system Linearization2/F-16 Vehicle Systems Model/Vehicle/LandingGear GroundReaction/Nose Gear Geometry Forces and Moments/GenerateGroundFM/LocMatrix1 ==
  note: 正負號可能相反
  note: $z_g^{B^{\prime } }$
  note: $x_g^B$
  note: ${\left\{\begin{array}{c} L_G =Y_G \cdot z_g^{B^{\prime } } -Z_G \cdot y_g^B \\ M_G =Z_G \cdot x_g^B -X_G \cdot z_g^{B^{\prime } } \\ N_G =X_G \cdot y_g^B -Y_G \cdot x_g^B \end{array}\right)}={\left[\begin{array}{ccc} 0 & z_g^{B^{\prime } } & -y_g^B \\ -z_g^{B^{\prime } } & 0 & x_g^B \\ y_g^B & -x_g^B & 0 \end{array}\right]}{\left[\begin{array}{c} X_G \\ Y_G \\ Z_G \end{array}\right]}={\left[\begin{array}{ccc} A_{11} & A_{12} & A_{13} \\ A_{21} & A_{22} & A_{23} \\ A_{31} & A_{32} & A_{33} \end{array}\right]}{\left[\begin{array}{c} X_G \\ Y_G \\ Z_G \end{array}\right]}$
  note: 詹庭宇:HL-20 example建模正負號有誤
  note: $y_g^B$
  note: $z_g^B$
  XgB : Inport
  ZgB_prime : Inport  Port=2
  Create 3x3 Matrix : sharedutil/Create 3x3 Matrix  aMode=aMode
      settings: SourceProductBaseCode=AE,PW,DR,MT,VE
  Demux2 : Demux  Outputs=3
  Terminator1 : Terminator
  inv1 : Gain  Gain=-1
  inv3 : Gain  Gain=-1
  inv4 : Gain  Gain=-1
  zero1 : Constant  Value=0  SampleTime=0
  zero2 : Constant  Value=0  SampleTime=0
  zero3 : Constant  Value=0  SampleTime=0
  A : Outport
  wires:
  XgB/1 -> Demux2/1
  Create 3x3 Matrix/1 -> A/1
  zero1/1 -> Create 3x3 Matrix/1
  Demux2/3 -> Terminator1/1
  ZgB_prime/1 -> Create 3x3 Matrix/2, inv4/1
  zero2/1 -> Create 3x3 Matrix/5
  zero3/1 -> Create 3x3 Matrix/9
  Demux2/2 -> Create 3x3 Matrix/7, inv1/1
  Demux2/1 -> Create 3x3 Matrix/6, inv3/1
  inv1/1 -> Create 3x3 Matrix/3
  inv4/1 -> Create 3x3 Matrix/4
  inv3/1 -> Create 3x3 Matrix/8

== system Linearization2/F-16 Vehicle Systems Model/Vehicle/LandingGear GroundReaction/Nose Gear Geometry Forces and Moments/GenerateGroundFM/Rotation Speed(TVC ON) ==
  friction : Inport
  In Bus Element38 : Inport  Port=2  PortName=PlantData  Element=Vt
  Gain1 : Gain  Gain=0.1
  Gain2 : Gain  Gain=0.5
  Switch : Switch  Threshold=180  SaturateOnIntegerOverflow=off  InputSameDT=off
  output : Outport
  wires:
  In Bus Element38/1 -> Switch/2
  friction/1 -> Gain1/1, Gain2/1
  Switch/1 -> output/1
  Gain2/1 -> Switch/3
  Gain1/1 -> Switch/1

== system Linearization2/F-16 Vehicle Systems Model/Vehicle/LandingGear GroundReaction/R Main Gear Geometry Forces and Moments/Calc Gear Force and Pos/Subsystem ==
  note: 地面正向力(慣性座標)
  note: $N=F_{strut} /C_{33}$
  note: $F_{strut} =K{\left(∆z_g^B \right)}+C{\left(∆{\dot{z} }_g^B \right)}$
      | 支柱上的作用力(體座標)
  note: $∆{\dot{z} }_g^B$
  note: 定義：
      | 慣性座標+Z軸朝下
      | 體座標+Z軸朝下
  deltaZgB : Inport
  C33 : Inport  Port=2
  DampingConstant_N/m/sec1 : Gain  Gain=LandingGear.RM.DampingConstant
  NormalForce : Product  Inputs=*/  RndMeth=Zero
  SpringConstant_N/m1 : Gain  Gain=LandingGear.RM.SpringConstant
  Sum2 : Sum
  Xcmpr_prev : Memory  InheritSampleTime=on
  dCompression : Sum  Inputs=+-
  ground only pushes : Saturate  UpperLimit=inf  LowerLimit=0
  reaction : Gain  Gain=-1
  dZ_strut : Outport
  Fn_strut : Outport  Port=2
  wires:
  deltaZgB/1 -> Xcmpr_prev/1, dCompression/1, SpringConstant_N/m1/1, dZ_strut/1
  dCompression/1 -> DampingConstant_N/m/sec1/1
  DampingConstant_N/m/sec1/1 -> Sum2/2
  SpringConstant_N/m1/1 -> Sum2/1
  Sum2/1 -> NormalForce/1  "Fstrut"
  NormalForce/1 -> ground only pushes/1
  ground only pushes/1 -> reaction/1
  reaction/1 -> Fn_strut/1
  Xcmpr_prev/1 -> dCompression/2
  C33/1 -> NormalForce/2

== system Linearization2/F-16 Vehicle Systems Model/Vehicle/LandingGear GroundReaction/R Main Gear Geometry Forces and Moments/GenerateGroundFM/Forces and distances to LMN ==
  Fb : Inport
  Xg_gnd : Inport  Port=2
  force to moment : Product  Multiplication=Matrix(*)  InputSameDT=on  SaturateOnIntegerOverflow=on  OutDataTypeStr=Inherit: Same as first input
  transpose : Reshape  OutputDimensionality=Row vector (2-D)  OutputDimensions=[1,3]
  transpose1 : Reshape  OutputDimensionality=Column vector (2-D)  OutputDimensions=[1,3]
  LMNe : Outport
  wires:
  Fb/1 -> transpose/1
  transpose/1 -> force to moment/1
  Xg_gnd/1 -> force to moment/2
  force to moment/1 -> transpose1/1
  transpose1/1 -> LMNe/1

== system Linearization2/F-16 Vehicle Systems Model/Vehicle/LandingGear GroundReaction/R Main Gear Geometry Forces and Moments/GenerateGroundFM/LocMatrix1 ==
  note: 正負號可能相反
  note: $z_g^{B^{\prime } }$
  note: $x_g^B$
  note: ${\left\{\begin{array}{c} L_G =Y_G \cdot z_g^{B^{\prime } } -Z_G \cdot y_g^B \\ M_G =Z_G \cdot x_g^B -X_G \cdot z_g^{B^{\prime } } \\ N_G =X_G \cdot y_g^B -Y_G \cdot x_g^B \end{array}\right)}={\left[\begin{array}{ccc} 0 & z_g^{B^{\prime } } & -y_g^B \\ -z_g^{B^{\prime } } & 0 & x_g^B \\ y_g^B & -x_g^B & 0 \end{array}\right]}{\left[\begin{array}{c} X_G \\ Y_G \\ Z_G \end{array}\right]}={\left[\begin{array}{ccc} A_{11} & A_{12} & A_{13} \\ A_{21} & A_{22} & A_{23} \\ A_{31} & A_{32} & A_{33} \end{array}\right]}{\left[\begin{array}{c} X_G \\ Y_G \\ Z_G \end{array}\right]}$
  note: 詹庭宇:HL-20 example建模正負號有誤
  note: $y_g^B$
  note: $z_g^B$
  XgB : Inport
  ZgB_prime : Inport  Port=2
  Create 3x3 Matrix : sharedutil/Create 3x3 Matrix  aMode=aMode
      settings: SourceProductBaseCode=AE,PW,DR,MT,VE
  Demux2 : Demux  Outputs=3
  Terminator1 : Terminator
  inv1 : Gain  Gain=-1
  inv3 : Gain  Gain=-1
  inv4 : Gain  Gain=-1
  zero1 : Constant  Value=0  SampleTime=0
  zero2 : Constant  Value=0  SampleTime=0
  zero3 : Constant  Value=0  SampleTime=0
  A : Outport
  wires:
  XgB/1 -> Demux2/1
  Create 3x3 Matrix/1 -> A/1
  zero1/1 -> Create 3x3 Matrix/1
  Demux2/3 -> Terminator1/1
  ZgB_prime/1 -> Create 3x3 Matrix/2, inv4/1
  zero2/1 -> Create 3x3 Matrix/5
  zero3/1 -> Create 3x3 Matrix/9
  Demux2/2 -> Create 3x3 Matrix/7, inv1/1
  Demux2/1 -> Create 3x3 Matrix/6, inv3/1
  inv1/1 -> Create 3x3 Matrix/3
  inv4/1 -> Create 3x3 Matrix/4
  inv3/1 -> Create 3x3 Matrix/8

== system Linearization2/F-16 Vehicle Systems Model/Vehicle/LandingGear GroundReaction/R Main Gear Geometry Forces and Moments/GenerateGroundFM/Rotation Speed(TVC ON) ==
  friction : Inport
  In Bus Element38 : Inport  Port=2  PortName=PlantData  Element=Vt
  Gain1 : Gain  Gain=0.1
  Gain2 : Gain  Gain=0.5
  Switch : Switch  Threshold=180  SaturateOnIntegerOverflow=off  InputSameDT=off
  output : Outport
  wires:
  In Bus Element38/1 -> Switch/2
  friction/1 -> Gain1/1, Gain2/1
  Switch/1 -> output/1
  Gain2/1 -> Switch/3
  Gain1/1 -> Switch/1

== matlab function Linearization2/F-16 Vehicle Systems Model/μαβ NDI Controller/attitude NDI ==
  data: y_bar input; p_c output; g2 input; q_c output; r_c output
function [p_c, q_c, r_c] = NDI(y_bar, g2)

u_bar = g2 \ y_bar;
% u_bar =pinv(g_s)*y_bar;     
p_c = u_bar(1);
q_c = u_bar(2);
r_c = u_bar(3);


end

== matlab function Linearization2/F-16 Vehicle Systems Model/Vehicle/6DOF (Quaternion)/Quateration ==
  data: Q input; phi output; theta output; psi output
function [phi,theta,psi] =Quateration(Q)

q0 = Q(1);
q1 = Q(2);
q2 = Q(3);
q3 = Q(4);

%% phi
phi_a = (2*(q0*q1+q2*q3));
phi_b = (q0.^2-q1.^2-q2.^2+q3.^2);
phi = atan2(phi_a,phi_b);%rad
% if phi>180
%     phi = 360-abs(phi);
% end
%% theta
theta = asin((2*q0*q2)-(2*q3*q1));%rad
% psi = atan((2*(q0*q3+q1*q2))/(q0.^2+q1.^2-q2.^2-q3.^2));%rad
% phi = atan((2*(q0*q1+q2*q3))/(q0.^2-q1.^2-q2.^2+q3.^2));%rad
%% psi
psi_a = (2*(q0*q3+q1*q2));
psi_b = (q0.^2+q1.^2-q2.^2-q3.^2);
psi = atan2(psi_a,psi_b);%rad
% if psi>180
%     psi = 360-abs(psi);
% end
%%
%test q0^2+q1^2+q2^2+Q3^3=1
% test = q0.^2+q1.^2+q2.^2+q3.^2;
% Quater = [phi theta psi test];

% Quater=zeros(1,4);
% Quater(1)= phi;
% Quater(2)= theta;
% Quater(3)= psi;
% Quater(4)= test;
end

== matlab function Linearization2/Environment/ISP /MATLAB Function ==
  data: h input; ISP_output output
function ISP_output =ISP(h)
%%  Symbol:
% a = Speed of sound.
% C = The temperature in Celsius.
% Cv = Constant volime ; Cv = e(internal energy)/T.
% Cp = Constant pressure ; Cp = h(enthalpy)/T.
% e = Internal energy.
% e_tr = Translational energy.
% e_rot = Rotational energy.
% e_vib = Vibrational energy.
% g = Is the gravitational acceleration at height h above sea level.
% go = Is the standard gravitational acceleration.
% gamma = Define Cp(constant pressure)/Cv(constant volime).
% h = Geometric altitude.
% mu = Coefficient of viscosity.
% P = The standard atmosphere at h.
% re = Is the Earth's mean radius.
% R = The gas constant for air.
% T = Is temperature in K.
% To = Is the sea_level temperature (absolute).
% rho = Density.
%% Gravitational acceleration 
go=9.806645;     % m/s^2
re=6356766;      % m
g=go*(re/(re+h))^2;
%%  Standard Atmosphere and Temperature
if h<11000 %11000m 以下
    P = (1013.25*(1-(2.25577e-5*h))^5.255879)*100 ;%unit Pa
    T = 288.15-((6.5e-3*h)); %unit K
elseif h ==11000
    P = 2.263203776117090e+04; %unit Pa
    T = 216.6500; %unit K
elseif h>11000 && h<20000 
    P = (226.32*exp(-0.000157688*(h-11000)) )*100; %unit Pa
    T = 216.6500; %unit K
elseif h==20000
    P = 5.474893557709153e+03; %unit Pa
    T = 216.6500; %unit K
else
    P = (54.7482*((1+4.61574e-6*(h-20000)))^-34.163215)*100 ; %unit Pa
    T = 216.6500+1e-3*(h-20000);%unit K
end
%%  Density
% The gas constant for air in SI units [(N*m)/(kg*K)].
R=287.0528;
rho=P/(R*T);
%%  Coefficient of viscosity
% Viscosity in SI units [kg/(s*m)].
mu=1.458*(10^-6)*((T^1.5)/(T+110.4));
%%  Speed of sound 
% molecular energy.
e_tr=(3/2)*R*T;
e_rot=R*T;
e_vib=(1/2)*R*T;
if ( T >= 600 ) % when the air temperature reaches 600K or higher .
    e=e_tr+e_rot+e_vib;
    Cv=e/T;
    Cp=(e+R*T)/T;
else
    e=e_tr+e_rot;
    Cv=e/T;
    Cp=(e+R*T)/T;
end
gamma=Cp/Cv;
% Speed of sound .
a=sqrt(gamma*R*T);
%%
ISP_output = [T,a,P,rho,g,mu];

== matlab function Linearization2/F-16 Vehicle Systems Model/Aerodynamic1/ISP /MATLAB Function ==
  data: h input; ISP_output output
function ISP_output =ISP(h)
%%  Symbol:
% a = Speed of sound.
% C = The temperature in Celsius.
% Cv = Constant volime ; Cv = e(internal energy)/T.
% Cp = Constant pressure ; Cp = h(enthalpy)/T.
% e = Internal energy.
% e_tr = Translational energy.
% e_rot = Rotational energy.
% e_vib = Vibrational energy.
% g = Is the gravitational acceleration at height h above sea level.
% go = Is the standard gravitational acceleration.
% gamma = Define Cp(constant pressure)/Cv(constant volime).
% h = Geometric altitude.
% mu = Coefficient of viscosity.
% P = The standard atmosphere at h.
% re = Is the Earth's mean radius.
% R = The gas constant for air.
% T = Is temperature in K.
% To = Is the sea_level temperature (absolute).
% rho = Density.
%% Gravitational acceleration 
go=9.806645;     % m/s^2
re=6356766;      % m
g=go*(re/(re+h))^2;
%%  Standard Atmosphere and Temperature
if h<11000 %11000m 以下
    P = (1013.25*(1-(2.25577e-5*h))^5.255879)*100 ;%unit Pa
    T = 288.15-((6.5e-3*h)); %unit K
elseif h ==11000
    P = 2.263203776117090e+04; %unit Pa
    T = 216.6500; %unit K
elseif h>11000 && h<20000 
    P = (226.32*exp(-0.000157688*(h-11000)) )*100; %unit Pa
    T = 216.6500; %unit K
elseif h==20000
    P = 5.474893557709153e+03; %unit Pa
    T = 216.6500; %unit K
else
    P = (54.7482*((1+4.61574e-6*(h-20000)))^-34.163215)*100 ; %unit Pa
    T = 216.6500+1e-3*(h-20000);%unit K
end
%%  Density
% The gas constant for air in SI units [(N*m)/(kg*K)].
R=287.0528;
rho=P/(R*T);
%%  Coefficient of viscosity
% Viscosity in SI units [kg/(s*m)].
mu=1.458*(10^-6)*((T^1.5)/(T+110.4));
%%  Speed of sound 
% molecular energy.
e_tr=(3/2)*R*T;
e_rot=R*T;
e_vib=(1/2)*R*T;
if ( T >= 600 ) % when the air temperature reaches 600K or higher .
    e=e_tr+e_rot+e_vib;
    Cv=e/T;
    Cp=(e+R*T)/T;
else
    e=e_tr+e_rot;
    Cv=e/T;
    Cp=(e+R*T)/T;
end
gamma=Cp/Cv;
% Speed of sound .
a=sqrt(gamma*R*T);
%%
ISP_output = [T,a,P,rho,g,mu];
